simulink model "LCK_old"  (R2018b)
settings: Solver=FixedStepDiscrete  StartTime=0.0  StopTime=inf  FixedStep=0.005  RelTol=1e-3
PostLoadFcn:
  | if any(exist('dsrtsu_mdlpostloadfcn', 'file') ~= 0), dsrtsu_mdlpostloadfcn('Execute', bdroot); end
values from neighbouring files (symbols this model uses):
  C_DEG2RAD = 0.0175    [LCK_Macro.sldd]
  C_KPH2MPS = 0.2778    [LCK_Macro.sldd]
  C_NEARZERO = 0.0001    [LCK_Macro.sldd]
  C_ONE = 1.0    [LCK_Macro.sldd]
  C_RAD2DEG = 57.2958    [LCK_Macro.sldd]
  C_ZERO = 0.0    [LCK_Macro.sldd]
  k_accel_pedal_pos_per_speed_x : value not decoded    [LCK_LogicPara.sldd]
  k_accel_pedal_pos_per_speed_z : value not decoded    [LCK_LogicPara.sldd]
  k_brake_suprress_hold = 1000.0    [LCK_LogicPara.sldd]
  k_driver_appl_torque_filt = 50.0    [LCK_LogicPara.sldd]
  k_driver_suppression_hold_time = 3000.0    [LCK_LogicPara.sldd]
  k_hands_on_wheel_hold_msec = 500.0    [LCK_LogicPara.sldd]
  k_hands_on_wheel_torque_hi = 0.2    [LCK_LogicPara.sldd]
  k_hands_on_wheel_torque_lo = 0.15    [LCK_LogicPara.sldd]
  k_handsoff_delay_cycles = 50.0    [LCK_LogicPara.sldd]
  k_handsoff_torq_Lo_CR = 0.3    [LCK_LogicPara.sldd]
  k_handson_delay_cycles = 5.0    [LCK_LogicPara.sldd]
  k_HighAccel_suppress_hold = 3000.0    [LCK_LogicPara.sldd]
  k_HLR_suprress_hold = 3000.0    [LCK_LogicPara.sldd]
  k_hs_StrAng_CR_threshold_z : value not decoded    [LCK_LogicPara.sldd]
  k_LC_Exit_Switch = 0.0    [LCK_LogicPara.sldd]
  k_LCG_Configured = 1.0    [LCK_LogicPara.sldd]
  k_LCK_A0_Rdy2Act_UseConst = 0.0    [LCK_LogicPara.sldd]
  k_LCK_A0Fac_ActSta : value not decoded    [LCK_CtrlPara.sldd]
  k_LCK_A0Fac_DrvStm : value not decoded    [LCK_CtrlPara.sldd]
  k_LCK_A0Shift_LftCurv : value not decoded    [LCK_CtrlPara.sldd]
  k_LCK_A0Shift_RgtCurv : value not decoded    [LCK_CtrlPara.sldd]
  k_LCK_A0Shift_StraLan = 0.0    [LCK_CtrlPara.sldd]
  k_LCK_A0ShiftFac_Dy_LftCurv : value not decoded    [LCK_CtrlPara.sldd]
  k_LCK_A0ShiftFac_Dy_RgtCurv : value not decoded    [LCK_CtrlPara.sldd]
  k_LCK_A0ShiftFac_Vspd : value not decoded    [LCK_CtrlPara.sldd]
  k_LCK_accel_inhibit_thold = 35.0    [LCK_LogicPara.sldd]
  k_LCK_Active2Ready_Mask = 255.0    [LCK_LogicPara.sldd]
  k_LCK_CvatRateBks : value not decoded    [LCK_CtrlPara.sldd]
  k_LCK_CvatrBks : value not decoded    [LCK_CtrlPara.sldd]
  k_LCK_DFac_Dy : value not decoded    [LCK_CtrlPara.sldd]
  k_LCK_DFac_Dy_Curv : value not decoded    [LCK_CtrlPara.sldd]
  k_LCK_DFac_HaCurCen : value not decoded    [LCK_CtrlPara.sldd]
  k_LCK_DFac_HaCurSid : value not decoded    [LCK_CtrlPara.sldd]
  k_LCK_DFac_HadCurCen : value not decoded    [LCK_CtrlPara.sldd]
  k_LCK_DFac_HadCurSid : value not decoded    [LCK_CtrlPara.sldd]
  k_LCK_DFac_HadStrCen : value not decoded    [LCK_CtrlPara.sldd]
  k_LCK_DFac_HadStrSid : value not decoded    [LCK_CtrlPara.sldd]
  k_LCK_DFac_HaStrCen : value not decoded    [LCK_CtrlPara.sldd]
  k_LCK_DFac_HaStrSid : value not decoded    [LCK_CtrlPara.sldd]
  k_LCK_DFac_Rad : value not decoded    [LCK_CtrlPara.sldd]
  k_LCK_DFac_SA_CurCen : value not decoded    [LCK_CtrlPara.sldd]
  k_LCK_DFac_SA_CurSid : value not decoded    [LCK_CtrlPara.sldd]
  k_LCK_DFac_SA_StrCen : value not decoded    [LCK_CtrlPara.sldd]
  k_LCK_DFac_SA_StrSid : value not decoded    [LCK_CtrlPara.sldd]
  k_LCK_DFac_SS_CurCen : value not decoded    [LCK_CtrlPara.sldd]
  k_LCK_DFac_SS_CurSid : value not decoded    [LCK_CtrlPara.sldd]
  k_LCK_DFac_SS_StrCen : value not decoded    [LCK_CtrlPara.sldd]
  k_LCK_DFac_SS_StrSid : value not decoded    [LCK_CtrlPara.sldd]
  k_LCK_DFac_Vspd : value not decoded    [LCK_CtrlPara.sldd]
  k_LCK_DlyTm_DrvStim = 0.2    [LCK_CtrlPara.sldd]
  k_LCK_DTermMax = 2.0    [LCK_CtrlPara.sldd]
  k_LCK_DyBks_Curv : value not decoded    [LCK_CtrlPara.sldd]
  k_LCK_Enable_POOnly = 1.0    [LCK_LogicPara.sldd]
  k_LCK_Entry_DistBuffer = 0.1    [LCK_LogicPara.sldd]
  k_LCK_Fac_Vspd2RngThr_FalRec = 0.23    [LCK_CtrlPara.sldd]
  k_LCK_Ffw_CvatSwh = 0.0    [LCK_CtrlPara.sldd]
  k_LCK_Ffw_DyBks : value not decoded    [LCK_CtrlPara.sldd]
  k_LCK_Ffw_TimCon_CmdFlt = 0.0    [LCK_CtrlPara.sldd]
  k_LCK_FfwDeltaFac_Rad_Lft : value not decoded    [LCK_CtrlPara.sldd]
  k_LCK_FfwDeltaFac_Rad_Rgt : value not decoded    [LCK_CtrlPara.sldd]
  k_LCK_FfwDeltaFac_Vspd : value not decoded    [LCK_CtrlPara.sldd]
  k_LCK_FfwFac_CvatRate_Lft : value not decoded    [LCK_CtrlPara.sldd]
  k_LCK_FfwFac_CvatRate_Rgt : value not decoded    [LCK_CtrlPara.sldd]
  k_LCK_FfwFac_Dy : value not decoded    [LCK_CtrlPara.sldd]
  k_LCK_FfwFac_Rad_Lft : value not decoded    [LCK_CtrlPara.sldd]
  k_LCK_FfwFac_Rad_Rgt : value not decoded    [LCK_CtrlPara.sldd]
  k_LCK_FfwFac_Vspd : value not decoded    [LCK_CtrlPara.sldd]
  k_LCK_FfwTorq_Cvat : value not decoded    [LCK_CtrlPara.sldd]
  k_LCK_HAFac_ActSta : value not decoded    [LCK_CtrlPara.sldd]
  k_LCK_HAFac_DrvStm : value not decoded    [LCK_CtrlPara.sldd]
  k_LCK_HaloTime = 2000.0    [LCK_LogicPara.sldd]
  k_LCK_HaloTime_Switch = 0.0    [LCK_LogicPara.sldd]
  k_LCK_HARFac_ActSta : value not decoded    [LCK_CtrlPara.sldd]
  k_LCK_HARFac_DrvStm : value not decoded    [LCK_CtrlPara.sldd]
  k_LCK_Hed_DyBks : value not decoded    [LCK_CtrlPara.sldd]
  k_LCK_HedAngDiffX : value not decoded    [LCK_CtrlPara.sldd]
  k_LCK_HedAngRateDiffX : value not decoded    [LCK_CtrlPara.sldd]
  k_LCK_HndsOnWhel_DlyTm_Idl2Rdy = 0.0    [LCK_LogicPara.sldd]
  k_LCK_host_veh_width = 1.86    [LCK_LogicPara.sldd]
  k_LCK_Idle2Ready_Mask = 239.0    [LCK_LogicPara.sldd]
  k_LCK_Junc_SusTime = 1.0    [LCK_LogicPara.sldd]
  k_LCK_KpKdDecSlopeLmt = 10.0    [LCK_CtrlPara.sldd]
  k_LCK_KpKdIncSlopeLmt = 5.0    [LCK_CtrlPara.sldd]
  k_LCK_Lat_Ctrl_DFac_Lft = 1.0    [LCK_CtrlPara.sldd]
  k_LCK_Lat_Ctrl_DFac_Rgt = 1.05    [LCK_CtrlPara.sldd]
  k_LCK_Lat_Ctrl_Kd = 0.8    [LCK_CtrlPara.sldd]
  k_LCK_Lat_Ctrl_Ki = 0.5    [LCK_CtrlPara.sldd]
  k_LCK_Lat_Ctrl_Kp = 0.7    [LCK_CtrlPara.sldd]
  k_LCK_Lat_Ctrl_Kp_NearGain = 0.7    [LCK_CtrlPara.sldd]
  k_LCK_Lat_Ctrl_PFac_Lft = 1.0    [LCK_CtrlPara.sldd]
  k_LCK_Lat_Ctrl_PFac_Rgt = 1.05    [LCK_CtrlPara.sldd]
  k_LCK_Lat_Ctrl_TimCon_CmdFlt = 5.0    [LCK_CtrlPara.sldd]
  k_LCK_Lat_DFac_Rad : value not decoded    [LCK_CtrlPara.sldd]
  k_LCK_Lat_DFac_SS_Cur : value not decoded    [LCK_CtrlPara.sldd]
  k_LCK_Lat_DFac_SS_Str : value not decoded    [LCK_CtrlPara.sldd]
  k_LCK_Lat_DFac_Vspd : value not decoded    [LCK_CtrlPara.sldd]
  k_LCK_Lat_DyBks : value not decoded    [LCK_CtrlPara.sldd]
  k_LCK_Lat_IFac_Rad : value not decoded    [LCK_CtrlPara.sldd]
  k_LCK_Lat_IFac_Vspd : value not decoded    [LCK_CtrlPara.sldd]
  k_LCK_Lat_ILmtFac_Dy_CurvLan : value not decoded    [LCK_CtrlPara.sldd]
  k_LCK_Lat_ILmtFac_Dy_StraLan : value not decoded    [LCK_CtrlPara.sldd]
  k_LCK_Lat_ILmtFac_Rad : value not decoded    [LCK_CtrlPara.sldd]
  k_LCK_Lat_ILmtFac_Rad_NearGain = 1.0    [LCK_CtrlPara.sldd]
  k_LCK_Lat_ILmtFac_Vspd_CurvLan : value not decoded    [LCK_CtrlPara.sldd]
  k_LCK_Lat_ILmtFac_Vspd_StraLan : value not decoded    [LCK_CtrlPara.sldd]
  k_LCK_Lat_ITermLmt_Dy = 1.0    [LCK_CtrlPara.sldd]
  k_LCK_Lat_KpKdDecSlopeLmt = 10.0    [LCK_CtrlPara.sldd]
  k_LCK_Lat_KpKdIncSlopeLmt = 10.0    [LCK_CtrlPara.sldd]
  k_LCK_Lat_PFac_Dy_InnLftCur : value not decoded    [LCK_CtrlPara.sldd]
  k_LCK_Lat_PFac_Dy_InnRgtCur : value not decoded    [LCK_CtrlPara.sldd]
  k_LCK_Lat_PFac_Dy_OutLftCur : value not decoded    [LCK_CtrlPara.sldd]
  k_LCK_Lat_PFac_Dy_OutRgtCur : value not decoded    [LCK_CtrlPara.sldd]
  k_LCK_Lat_PFac_Dy_Str : value not decoded    [LCK_CtrlPara.sldd]
  k_LCK_Lat_PFac_Rad : value not decoded    [LCK_CtrlPara.sldd]
  ... (+158 more)
undefined symbols (not defined in the file or in its folder): k_LCK_CurvBks, K_LCK_SPA0A1A2_LMRngCmp_y
libraries: LateralControl_fcns_lib x58, simulink x22
(part 42 of 45)

== stateflow chart LCK_old/Lateral_Control_Module/Adas_Lateral_Control_LCK_Core/Module 3/Sig_Wekng_0/Trigger Hold Counter/Trigger Hold ==
  settings: description=_GWMH9P5.LCK.111_13_
  (default) -> (junction 11)
  (junction 11) -> (junction 13) [order 1] : [(Trigger==1)]...
      | {count = 0;}
  (junction 11) -> (junction 14) [order 2]
  (junction 13) -> (junction 17)
  (junction 14) -> (junction 17) [order 1] : [count<= hold_time]
  (junction 14) -> (junction 15) [order 2] : {Out = 0;}
  (junction 17) -> (junction 16) : {
      | Out = 1;...
      | count = count + ML_TIME_MSEC;
      | }
  (junction 15) -> (junction 16)
  (junction 16) -> (junction 25)
  data: Trigger input [0..1]; hold_time input; Out output boolean [0..1]; count output single; ML_TIME_MSEC parameter single
  data Trigger settings: description=_GWMH9P5.LCK.111_116_
  data hold_time settings: description=_GWMH9P5.LCK.111_117_
  data Out settings: description=|
      | _GACA26P4.LCK.111_66_
      | $TL$ type=Bool; date=20190416T145812; $TL$
  data count settings: description=|
      | _GACA26P4.LCK.111_67_
      | $TL$ type=Float32; date=20190416T145816; $TL$
  data ML_TIME_MSEC settings: description=|
      | _GACA26P4.LCK.111_68_
      | $TL$ name=$O; type=ESR_Typedefs/unsigned8_T; class=EXTERN_MACRO; date=20190416T150613; $TL$

== stateflow chart LCK_old/Main_OS ==
  settings: updateMethod=DISCRETE  sampleTime=0.005
  note: 5 ms
      | loop
  note: 20 ms
      | loop
  (default) -> (junction 9)
  (junction 9) -> (junction 10) : {
      | do_VehSig2EyeQ_Tx_5ms;
      |
      | }
  (junction 10) -> (junction 13) [order 1] : [ i == 3]
  (junction 10) -> (junction 11) [order 2] : {
      | i = i + 1;
      | }
  (junction 13) -> (junction 12) : {
      | do_Lateral_Control_20ms;
      | do_Lat_Ctrl_Tx_20ms;
      | i = 0;
      | }
  (junction 11) -> (junction 12)
  (junction 12) -> (junction 22) : {
      |
      | }
  data: i local double
  events: do_Lateral_Control_20ms output FUNCTION_CALL_EVENT; do_Lat_Ctrl_Tx_20ms output FUNCTION_CALL_EVENT; do_VehSig2EyeQ_Tx_5ms output FUNCTION_CALL_EVENT

== stateflow chart LCK_old/Lateral_Control_Module/LC_Path_Process/Chart ==
  state LC_Phase3
    en:
    LC_Phase = 3;
  state LC_Phase1
    en:
    LC_Phase = 1;
  state Initialization
    en:
    LC_Phase = 0;
  state LC_Phase4
    en:
    LC_Phase = 4;
  state LC_Phase2
    en:
    LC_Phase = 2;
  Initialization -> LC_Phase3 [order 2] : [LCK_Mode==6]
  Initialization -> LC_Phase1 [order 1] : [LCK_Mode==5]
  LC_Phase3 -> Initialization [order 1] : [(LCK_Mode~=5)&(LCK_Mode~=6)]
  LC_Phase1 -> Initialization [order 1] : [(LCK_Mode~=5)&(LCK_Mode~=6)]
  LC_Phase4 -> LC_Phase3 [order 2] : [(SPP_A0-SPP_A0_Pre)<-1]
  LC_Phase3 -> LC_Phase4 [order 2] : [(SPP_A0-SPP_A0_Pre)>1]
  LC_Phase1 -> LC_Phase2 [order 2] : [(SPP_A0-SPP_A0_Pre)<-1]
  LC_Phase2 -> LC_Phase1 [order 2] : [(SPP_A0-SPP_A0_Pre)>1]
  LC_Phase4 -> Initialization [order 1] : [(LCK_Mode~=5)&(LCK_Mode~=6)]
  LC_Phase2 -> Initialization [order 1] : [(LCK_Mode~=5)&(LCK_Mode~=6)]
  (default) -> Initialization
  data: SPP_A0 input; SPP_A0_Pre input; LCK_Mode input; LC_Phase output single

== stateflow chart LCK_old/Lateral_Control_Module/LC_Path_Process/LC_Path_Planning/Chart1 ==
  state Init
    en:
    iter_cnt = 0;
    LC_path_gen_flag=0;
    pass_cnt = 0;
    long_s=0;
  state LC_Gen
    en:
    LC_path_gen_flag=1;
    iter_cnt = 0;
    pass_cnt = pass_cnt+1;
    long_s=0;
    du:
    LC_path_gen_flag=0;
    pass_cnt = pass_cnt+1;
  state LC_Flag_Clear
    en:
    LC_path_gen_flag=0;
    pass_cnt = pass_cnt+1;
    long_s=long_s+vspd*0.02;
    du:
    iter_cnt = iter_cnt+1;
    pass_cnt = pass_cnt+1;
    long_s=long_s+vspd*0.02;
  (default) -> Init
  Init -> LC_Gen : [LC_Active==1]
  LC_Gen -> Init [order 2] : [LC_Active==0]
  LC_Flag_Clear -> Init [order 2] : [LC_Active==0]
  LC_Gen -> LC_Flag_Clear [order 1] : [LC_path_gen_flag==1]
  LC_Flag_Clear -> LC_Gen [order 1] : [iter_cnt==LC_iter_num]
  data: LC_Active input; LC_path_gen_flag output single; iter_cnt local; pass_cnt output single; vspd input; long_s output single; LC_iter_num input
